simulink model "Eas_Integrated"  (R2021a)
settings: Solver=FixedStepDiscrete  StartTime=0.0  StopTime=inf  FixedStep=0.01  RelTol=1e-3
values from neighbouring files (symbols this model uses):
  Accelerator_Pedal_0 = 0.0    [DPF_Data_Dictionary.sldd]
  Adblue_Concentration_1 = 31.8    [Scr_Regeneration.sldd]
  Adblue_Concentration_2 = 33.2    [Scr_Regeneration.sldd]
  Adblue_Low_Level = 20.0    [Scr_Regeneration.sldd]
  Break_Pedal_0 = 0.0    [DPF_Data_Dictionary.sldd]
  Clutch_Pedal_0 = 0.0    [DPF_Data_Dictionary.sldd]
  Constant = 3.0    [Scr_Regeneration.sldd]
  Coolant_Temp_80 = 80.0    [DPF_Data_Dictionary.sldd]
  Crank_Angle_10 = 10.0    [DPF_Data_Dictionary.sldd]
  Crank_Angle_190 = 190.0    [DPF_Data_Dictionary.sldd]
  Crank_Angle_215 = 215.0    [DPF_Data_Dictionary.sldd]
  Crank_Angle_35 = 35.0    [DPF_Data_Dictionary.sldd]
  Crank_Angle_370 = 370.0    [DPF_Data_Dictionary.sldd]
  Crank_Angle_395 = 395.0    [DPF_Data_Dictionary.sldd]
  Crank_Angle_550 = 550.0    [DPF_Data_Dictionary.sldd]
  Crank_Angle_575 = 575.0    [DPF_Data_Dictionary.sldd]
  Dcrg_Press = 6.0    [Scr_Regeneration.sldd]
  DPF_Temp_Auto_250 = 250.0    [DPF_Data_Dictionary.sldd]
  DPF_Temp_Manual_200 = 200.0    [DPF_Data_Dictionary.sldd]
  Lamp_Off = 1.0    [Scr_Regeneration.sldd]
  Lamp_On = 0.0    [Scr_Regeneration.sldd]
  Nozzle_Area = 1.13E-6    [Scr_Regeneration.sldd]
  Nozzle_FlowRate = 0.099    [Scr_Regeneration.sldd]
  rpm_1500 = 1500.0    [DPF_Data_Dictionary.sldd]
  scr_temp200 = 200.0    [Scr_Regeneration.sldd]
  Soot_Deposition_Auto_80 = 80.0    [DPF_Data_Dictionary.sldd]
  Soot_Deposition_Manual_80 = 80.0    [DPF_Data_Dictionary.sldd]
  Soot_Deposition_Service_95 = 95.0    [DPF_Data_Dictionary.sldd]
  Tank_Condition = 0.0    [Scr_Regeneration.sldd]
  Var = 2.0    [Scr_Regeneration.sldd]
  Vehicle_Speed_55 = 55.0    [DPF_Data_Dictionary.sldd]
undefined symbols (not defined in the file or in its folder): adblue_capacity
libraries: simulink x2
settings Model: DataDictionary=DPF_Data_Dictionary.sldd  Creator=Admin  LastModifiedBy=SOMNATH
settings OptimizationCC: BlockReduction=off  DefaultParameterBehavior=Inlined  UseDivisionForNetSlopeComputation=on  EnhancedBackFolding=on  PassReuseOutputArgsAs=Individual arguments  EfficientFloat2IntCast=on  LifeSpan=Inf  OptimizeBlockOrder=speed  DifferentSizesBufferReuse=on  OptimizationCustomize=off  EfficientTunableParamExpr=on
settings DebuggingCC: SignalInfNanChecking=error  SignalRangeChecking=error  ReadBeforeWriteMsg=EnableAllAsError  WriteAfterWriteMsg=EnableAllAsError  WriteAfterReadMsg=EnableAllAsError  AlgebraicLoopMsg=error  ArtificialAlgebraicLoopMsg=error  SaveWithDisabledLinksMsg=error  SaveWithParameterizedLinksMsg=error  BlockPriorityViolationMsg=error  SolverPrmCheckMsg=error  InheritedTsInSrcMsg=error  SingleTaskRateTransMsg=error  TasksWithSamePriorityMsg=error  SigSpecEnsureSampleTimeMsg=error  CheckMatrixSingularityMsg=error  IntegerOverflowMsg=error  ParameterUnderflowMsg=error  ParameterPrecisionLossMsg=error  ParameterTunabilityLossMsg=error  UnderSpecifiedDataTypeMsg=error  UnnecessaryDatatypeConvMsg=warning  VectorMatrixConversionMsg=error  SignalLabelMismatchMsg=error  UnconnectedInputMsg=error  UnconnectedOutputMsg=error  UnconnectedLineMsg=error  SFcnCompatibilityMsg=error  UniqueDataStoreMsg=error  BusObjectLabelMismatch=error  RootOutportRequireBusObject=error  AssertControl=DisableAll  ModelReferenceIOMsg=error  ModelReferenceIOMismatchMessage=error  UnknownTsInhSupMsg=error  ModelReferenceDataLoggingMessage=error  StateNameClashWarn=warning  StrictBusMsg=ErrorOnBusTreatedAsVector  NonBusSignalsTreatedAsBus=error  SFInvalidInputDataAccessInChartInitDiag=error  SFTransitionOutsideNaturalParentDiag=error  SFUnreachableExecutionPathDiag=error  SFUndirectedBroadcastEventsDiag=error  SFTransitionActionBeforeConditionDiag=error  SFTemporalDelaySmallerThanSampleTimeDiag=error  SFSelfTransitionDiag=error  SFExecutionAtInitializationDiag=error  IntegerSaturationMsg=error
settings SFSimCC: CompileTimeRecursionLimit=0  EnableRuntimeRecursion=off  MATLABDynamicMemAlloc=off
settings RTWCC: SystemTargetFile=ert.tlc  GenCodeOnly=on  TemplateMakefile=ert_default_tmf  GenerateReport=on  Toolchain=MinGW64 | gmake (64-bit Windows)  IncludeHyperlinkInReport=on  LaunchReport=on  GenerateTraceInfo=on  GenerateTraceReport=on  GenerateTraceReportSl=on  GenerateTraceReportSf=on  GenerateTraceReportEml=on  GenerateWebview=on  GenerateCodeReplacementReport=on
settings CodeAppCC: ForceParamTrailComments=on  IgnoreCustomStorageClasses=off  OperatorAnnotations=on  SimulinkDataObjDesc=on  SFDataObjDesc=on  MATLABFcnDesc=on  MangleLength=4  InsertBlockDesc=on  ReqsInCode=on
settings ERTTargetCC: TargetLangStandard=C99 (ISO)  UtilityFuncGeneration=Shared location  GenerateSampleERTMain=on  IncludeMdlTerminateFcn=off  SuppressErrorStatus=on  SupportAbsoluteTime=off  SupportNonFinite=off  ParenthesesLevel=Maximum  CastingMode=Standards  GenerateSharedConstants=off  InlinedParameterPlacement=NonHierarchical  ERTCustomFileTemplate=example_file_process.tlc  PreserveExpressionOrder=on  EnableSignedLeftShifts=off  EnableSignedRightShifts=off
settings ConfigComp: CovMetricSettings=dcmwe  DVMode=PropertyProving  DVTestSuiteOptimization=Auto  DVDetectDeadLogic=on  DVDetectActiveLogic=on  DVDetectOutOfBounds=on  DVDetectInfNaN=on  DVDesignMinMaxCheck=on  DVDetectDSMAccessViolations=on  DVDetectHISMViolationsHisl_0002=on  DVDetectHISMViolationsHisl_0003=on  DVDetectHISMViolationsHisl_0004=on  DVDetectHISMViolationsHisl_0028=on  DVDetectBlockInputRangeViolations=on  DVSaveExpectedOutput=on  DVRandomizeNoEffectData=on  DVSaveHarnessModel=on

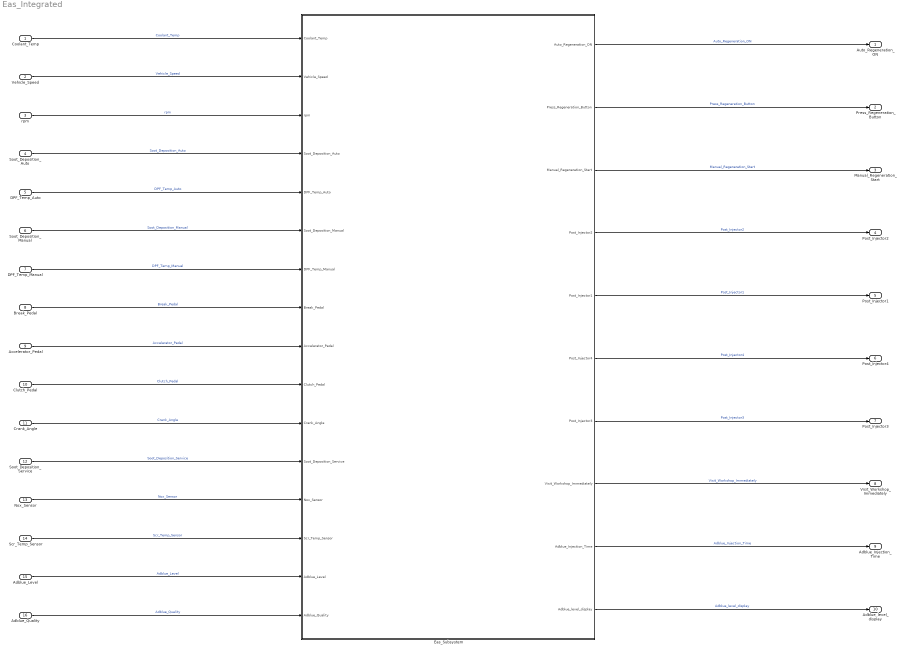
== system Eas_Integrated ==
  Coolant_Temp : Inport  OutDataTypeStr=int16
  Vehicle_Speed : Inport  Port=2  OutDataTypeStr=uint8
  rpm : Inport  Port=3  OutDataTypeStr=uint16
  Soot_Deposition_Auto : Inport  Port=4  OutDataTypeStr=uint8
  DPF_Temp_Auto : Inport  Port=5  OutDataTypeStr=uint8
  Soot_Deposition_Manual : Inport  Port=6  OutDataTypeStr=uint8
  DPF_Temp_Manual : Inport  Port=7  OutDataTypeStr=int16
  Break_Pedal : Inport  Port=8  OutDataTypeStr=boolean
  Accelerator_Pedal : Inport  Port=9  OutDataTypeStr=boolean
  Clutch_Pedal : Inport  Port=10  OutDataTypeStr=boolean
  Crank_Angle : Inport  Port=11  OutDataTypeStr=uint16
  Soot_Deposition_Service : Inport  Port=12  OutDataTypeStr=uint8
  Nox_Sensor : Inport  Port=13  OutDataTypeStr=uint16
  Scr_Temp_Sensor : Inport  Port=14  OutDataTypeStr=uint16
  Adblue_Level : Inport  Port=15  OutDataTypeStr=uint8
  Adblue_Quality : Inport  Port=16  OutDataTypeStr=double
  Eas_Subsystem : Subsystem  TreatAsAtomicUnit=on
  Auto_Regeneration_ON : Outport
  Press_Regeneration_Button : Outport  Port=2
  Manual_Regeneration_Start : Outport  Port=3
  Post_Injector2 : Outport  Port=4
  Post_Injector1 : Outport  Port=5
  Post_Injector4 : Outport  Port=6
  Post_Injector3 : Outport  Port=7
  Visit_Workshop_Immediately : Outport  Port=8
  Adblue_Injection_Time : Outport  Port=9  OutMin=0  OutMax=1500  OutDataTypeStr=double
  Adblue_level_display : Outport  Port=10  OutDataTypeStr=Enum: adblue_capacity
  wires:
  Eas_Subsystem/10(Adblue_level_display) -> Adblue_level_display/1  "Adblue_level_display"
  Eas_Subsystem/9(Adblue_Injection_Time) -> Adblue_Injection_Time/1  "Adblue_Injection_Time"
  Eas_Subsystem/7(Post_Injector3) -> Post_Injector3/1  "Post_Injector3"
  Eas_Subsystem/1(Auto_Regeneration_ON) -> Auto_Regeneration_ON/1  "Auto_Regeneration_ON"
  Eas_Subsystem/8(Visit_Workshop_Immediately) -> Visit_Workshop_Immediately/1  "Visit_Workshop_Immediately"
  Eas_Subsystem/6(Post_Injector4) -> Post_Injector4/1  "Post_Injector4"
  Eas_Subsystem/2(Press_Regeneration_Button) -> Press_Regeneration_Button/1  "Press_Regeneration_Button"
  Eas_Subsystem/5(Post_Injector1) -> Post_Injector1/1  "Post_Injector1"
  Eas_Subsystem/4(Post_Injector2) -> Post_Injector2/1  "Post_Injector2"
  Eas_Subsystem/3(Manual_Regeneration_Start) -> Manual_Regeneration_Start/1  "Manual_Regeneration_Start"
  Adblue_Quality/1 -> Eas_Subsystem/16(Adblue_Quality)  "Adblue_Quality"
  Adblue_Level/1 -> Eas_Subsystem/15(Adblue_Level)  "Adblue_Level"
  DPF_Temp_Auto/1 -> Eas_Subsystem/5(DPF_Temp_Auto)  "DPF_Temp_Auto"
  Accelerator_Pedal/1 -> Eas_Subsystem/9(Accelerator_Pedal)  "Accelerator_Pedal"
  Scr_Temp_Sensor/1 -> Eas_Subsystem/14(Scr_Temp_Sensor)  "Scr_Temp_Sensor"
  Nox_Sensor/1 -> Eas_Subsystem/13(Nox_Sensor)  "Nox_Sensor"
  Soot_Deposition_Service/1 -> Eas_Subsystem/12(Soot_Deposition_Service)  "Soot_Deposition_Service"
  Crank_Angle/1 -> Eas_Subsystem/11(Crank_Angle)  "Crank_Angle"
  Clutch_Pedal/1 -> Eas_Subsystem/10(Clutch_Pedal)  "Clutch_Pedal"
  Break_Pedal/1 -> Eas_Subsystem/8(Break_Pedal)  "Break_Pedal"
  DPF_Temp_Manual/1 -> Eas_Subsystem/7(DPF_Temp_Manual)  "DPF_Temp_Manual"
  Soot_Deposition_Manual/1 -> Eas_Subsystem/6(Soot_Deposition_Manual)  "Soot_Deposition_Manual"
  Soot_Deposition_Auto/1 -> Eas_Subsystem/4(Soot_Deposition_Auto)  "Soot_Deposition_Auto"
  rpm/1 -> Eas_Subsystem/3(rpm)  "rpm"
  Vehicle_Speed/1 -> Eas_Subsystem/2(Vehicle_Speed)  "Vehicle_Speed"
  Coolant_Temp/1 -> Eas_Subsystem/1(Coolant_Temp)  "Coolant_Temp"

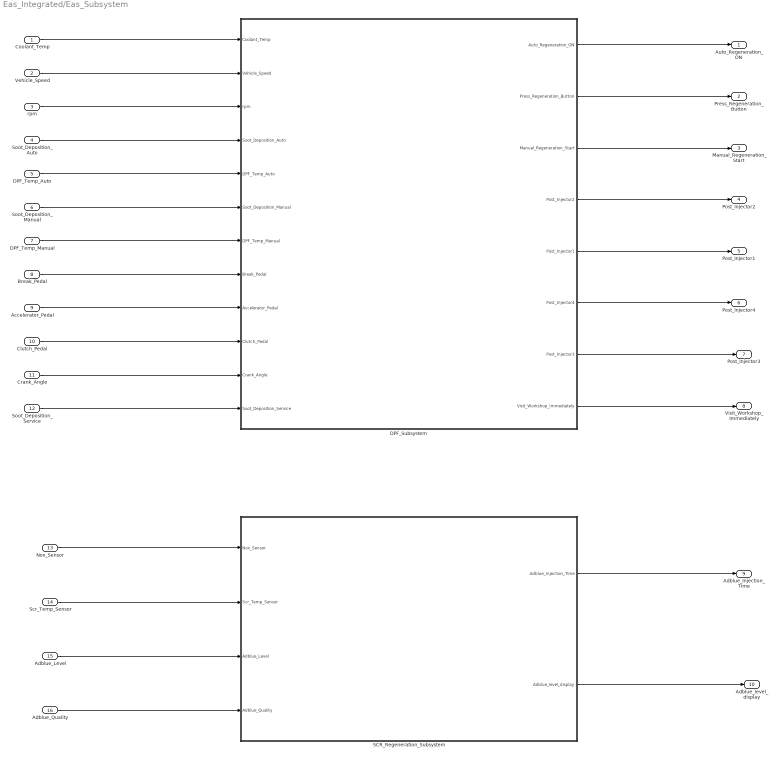
== system Eas_Integrated/Eas_Subsystem ==
  Coolant_Temp : Inport
  Vehicle_Speed : Inport  Port=2
  rpm : Inport  Port=3
  Soot_Deposition_Auto : Inport  Port=4
  DPF_Temp_Auto : Inport  Port=5
  Soot_Deposition_Manual : Inport  Port=6
  DPF_Temp_Manual : Inport  Port=7
  Break_Pedal : Inport  Port=8
  Accelerator_Pedal : Inport  Port=9
  Clutch_Pedal : Inport  Port=10
  Crank_Angle : Inport  Port=11
  Soot_Deposition_Service : Inport  Port=12
  Nox_Sensor : Inport  Port=13
  Scr_Temp_Sensor : Inport  Port=14
  Adblue_Level : Inport  Port=15  OutDataTypeStr=uint8
  Adblue_Quality : Inport  Port=16
  DPF_Subsystem : Subsystem  TreatAsAtomicUnit=on
  SCR_Regeneration_Subsystem : Subsystem  TreatAsAtomicUnit=on
  Auto_Regeneration_ON : Outport
  Press_Regeneration_Button : Outport  Port=2
  Manual_Regeneration_Start : Outport  Port=3
  Post_Injector2 : Outport  Port=4
  Post_Injector1 : Outport  Port=5
  Post_Injector4 : Outport  Port=6
  Post_Injector3 : Outport  Port=7
  Visit_Workshop_Immediately : Outport  Port=8
  Adblue_Injection_Time : Outport  Port=9
  Adblue_level_display : Outport  Port=10
  wires:
  Vehicle_Speed/1 -> DPF_Subsystem/2(Vehicle_Speed)
  SCR_Regeneration_Subsystem/1(Adblue_Injection_Time) -> Adblue_Injection_Time/1
  Accelerator_Pedal/1 -> DPF_Subsystem/9(Accelerator_Pedal)
  DPF_Temp_Manual/1 -> DPF_Subsystem/7(DPF_Temp_Manual)
  rpm/1 -> DPF_Subsystem/3(rpm)
  DPF_Temp_Auto/1 -> DPF_Subsystem/5(DPF_Temp_Auto)
  DPF_Subsystem/2(Press_Regeneration_Button) -> Press_Regeneration_Button/1
  Crank_Angle/1 -> DPF_Subsystem/11(Crank_Angle)
  Scr_Temp_Sensor/1 -> SCR_Regeneration_Subsystem/2(Scr_Temp_Sensor)
  Soot_Deposition_Auto/1 -> DPF_Subsystem/4(Soot_Deposition_Auto)
  DPF_Subsystem/5(Post_Injector1) -> Post_Injector1/1
  Soot_Deposition_Service/1 -> DPF_Subsystem/12(Soot_Deposition_Service)
  Soot_Deposition_Manual/1 -> DPF_Subsystem/6(Soot_Deposition_Manual)
  Adblue_Quality/1 -> SCR_Regeneration_Subsystem/4(Adblue_Quality)
  Clutch_Pedal/1 -> DPF_Subsystem/10(Clutch_Pedal)
  DPF_Subsystem/3(Manual_Regeneration_Start) -> Manual_Regeneration_Start/1
  Break_Pedal/1 -> DPF_Subsystem/8(Break_Pedal)
  DPF_Subsystem/7(Post_Injector3) -> Post_Injector3/1
  DPF_Subsystem/6(Post_Injector4) -> Post_Injector4/1
  Coolant_Temp/1 -> DPF_Subsystem/1(Coolant_Temp)
  DPF_Subsystem/8(Visit_Workshop_Immediately) -> Visit_Workshop_Immediately/1
  Nox_Sensor/1 -> SCR_Regeneration_Subsystem/1(Nox_Sensor)
  DPF_Subsystem/1(Auto_Regeneration_ON) -> Auto_Regeneration_ON/1
  DPF_Subsystem/4(Post_Injector2) -> Post_Injector2/1
  SCR_Regeneration_Subsystem/2(Adblue_level_display) -> Adblue_level_display/1
  Adblue_Level/1 -> SCR_Regeneration_Subsystem/3(Adblue_Level)

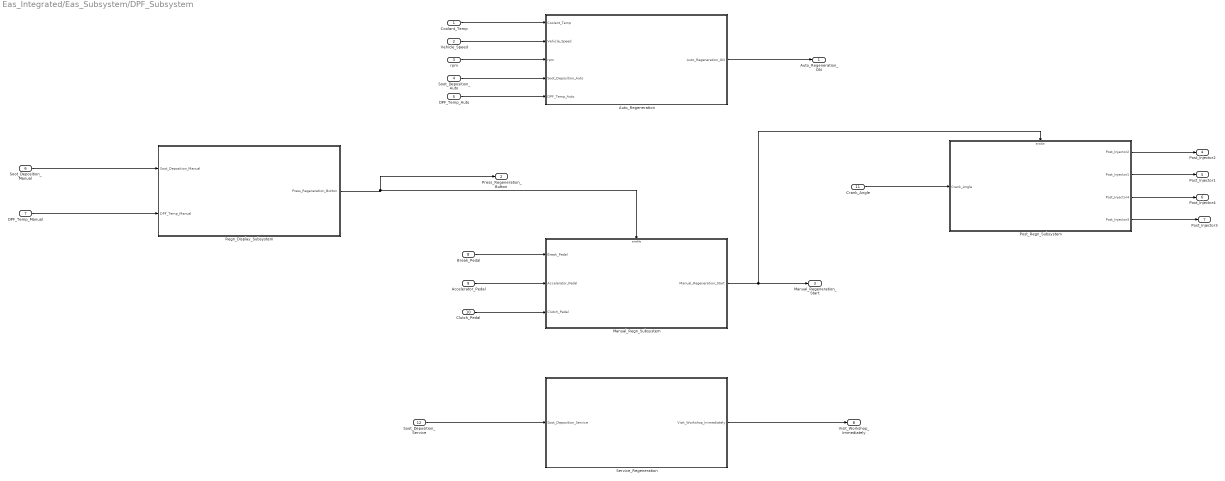
== system Eas_Integrated/Eas_Subsystem/DPF_Subsystem ==
  Coolant_Temp : Inport
  Vehicle_Speed : Inport  Port=2
  rpm : Inport  Port=3
  Soot_Deposition_Auto : Inport  Port=4
  DPF_Temp_Auto : Inport  Port=5
  Soot_Deposition_Manual : Inport  Port=6
  DPF_Temp_Manual : Inport  Port=7
  Break_Pedal : Inport  Port=8
  Accelerator_Pedal : Inport  Port=9
  Clutch_Pedal : Inport  Port=10
  Crank_Angle : Inport  Port=11
  Soot_Deposition_Service : Inport  Port=12
  Auto_Regeneration : Subsystem  TreatAsAtomicUnit=on
  Manual_Regn_Subsystem : Subsystem  TreatAsAtomicUnit=on
  Post_Regn_Subsystem : Subsystem
  Regn_Display_Subsystem : Subsystem
  Service_Regeneration : Subsystem
  Auto_Regeneration_ON : Outport
  Press_Regeneration_Button : Outport  Port=2
  Manual_Regeneration_Start : Outport  Port=3
  Post_Injector2 : Outport  Port=4
  Post_Injector1 : Outport  Port=5
  Post_Injector4 : Outport  Port=6
  Post_Injector3 : Outport  Port=7
  Visit_Workshop_Immediately : Outport  Port=8
  wires:
  Soot_Deposition_Auto/1 -> Auto_Regeneration/4(Soot_Deposition_Auto)
  Auto_Regeneration/1(Auto_Regeneration_ON) -> Auto_Regeneration_ON/1
  Coolant_Temp/1 -> Auto_Regeneration/1(Coolant_Temp)
  rpm/1 -> Auto_Regeneration/3(rpm)
  Vehicle_Speed/1 -> Auto_Regeneration/2(Vehicle_Speed)
  DPF_Temp_Auto/1 -> Auto_Regeneration/5(DPF_Temp_Auto)
  Crank_Angle/1 -> Post_Regn_Subsystem/1(Crank_Angle)
  Post_Regn_Subsystem/2(Post_Injector1) -> Post_Injector1/1
  Post_Regn_Subsystem/3(Post_Injector4) -> Post_Injector4/1
  Manual_Regn_Subsystem/1(Manual_Regeneration_Start) -> Manual_Regeneration_Start/1, Post_Regn_Subsystem/Enable
  Post_Regn_Subsystem/4(Post_Injector3) -> Post_Injector3/1
  Soot_Deposition_Manual/1 -> Regn_Display_Subsystem/1(Soot_Deposition_Manual)
  DPF_Temp_Manual/1 -> Regn_Display_Subsystem/2(DPF_Temp_Manual)
  Regn_Display_Subsystem/1(Press_Regeneration_Button) -> Manual_Regn_Subsystem/Enable, Press_Regeneration_Button/1
  Post_Regn_Subsystem/1(Post_Injector2) -> Post_Injector2/1
  Accelerator_Pedal/1 -> Manual_Regn_Subsystem/2(Accelerator_Pedal)
  Clutch_Pedal/1 -> Manual_Regn_Subsystem/3(Clutch_Pedal)
  Break_Pedal/1 -> Manual_Regn_Subsystem/1(Break_Pedal)
  Soot_Deposition_Service/1 -> Service_Regeneration/1(Soot_Deposition_Service)
  Service_Regeneration/1(Visit_Workshop_Immediately) -> Visit_Workshop_Immediately/1

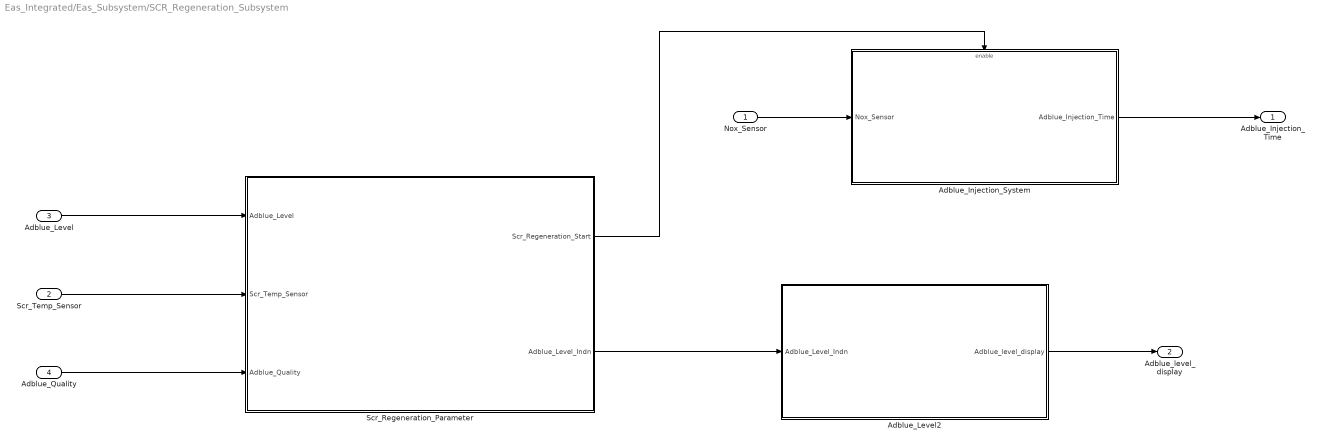
== system Eas_Integrated/Eas_Subsystem/SCR_Regeneration_Subsystem ==
  Nox_Sensor : Inport
  Scr_Temp_Sensor : Inport  Port=2
  Adblue_Level : Inport  Port=3  OutDataTypeStr=uint8
  Adblue_Quality : Inport  Port=4
  Adblue_Injection_System : Subsystem  Tag=Adblue_Injection_System
      settings: AttributesFormatString=%<Description>
  Adblue_Level2 : Subsystem  Tag=Adblue_Level2  Description=|  TreatAsAtomicUnit=on
      | This subsystem models a digital thermometer composed of a simple
      | temperature sensor and an ADC.
      settings: AttributesFormatString=%<Description>
  Scr_Regeneration_Parameter : Subsystem  Tag=Scr_Regeneration_Parameter  Description=|  TreatAsAtomicUnit=on
      | This subsystem models a digital thermometer composed of a simple
      | temperature sensor and an ADC.
      settings: AttributesFormatString=%<BlockDescription>
  Adblue_Injection_Time : Outport
  Adblue_level_display : Outport  Port=2
  wires:
  Scr_Regeneration_Parameter/1(Scr_Regeneration_Start) -> Adblue_Injection_System/Enable
  Adblue_Injection_System/1(Adblue_Injection_Time) -> Adblue_Injection_Time/1
  Scr_Temp_Sensor/1 -> Scr_Regeneration_Parameter/2(Scr_Temp_Sensor)
  Adblue_Level/1 -> Scr_Regeneration_Parameter/1(Adblue_Level)
  Scr_Regeneration_Parameter/2(Adblue_Level_Indn) -> Adblue_Level2/1(Adblue_Level_Indn)
  Nox_Sensor/1 -> Adblue_Injection_System/1(Nox_Sensor)
  Adblue_Level2/1(Adblue_level_display) -> Adblue_level_display/1
  Adblue_Quality/1 -> Scr_Regeneration_Parameter/3(Adblue_Quality)

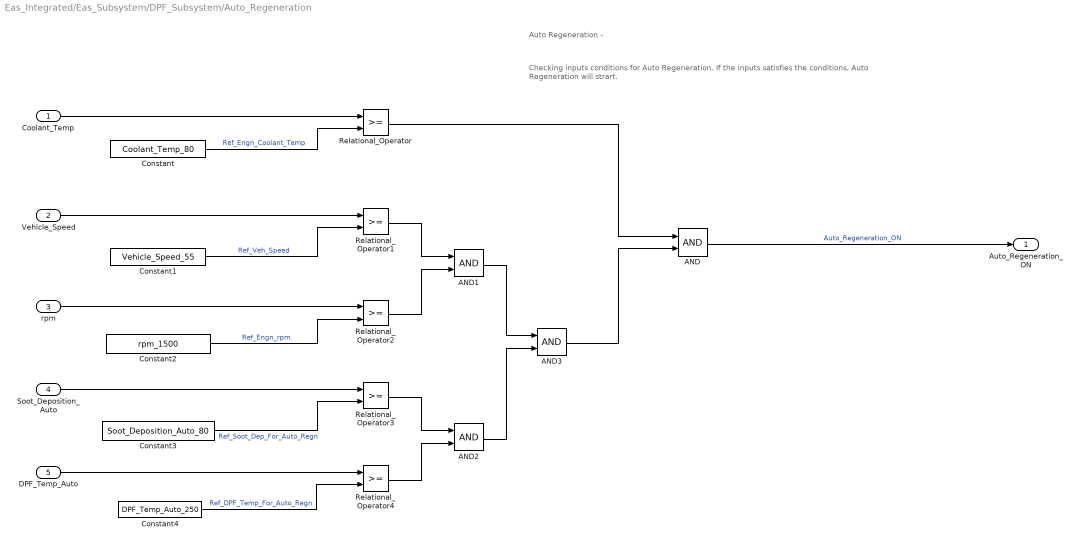
== system Eas_Integrated/Eas_Subsystem/DPF_Subsystem/Auto_Regeneration ==
  note: Auto Regeneration -
  note: Checking inputs conditions for Auto Regeneration. If the inputs satisfies the conditions, Auto Regeneration will strart.
  Coolant_Temp : Inport
  Vehicle_Speed : Inport  Port=2
  rpm : Inport  Port=3
  Soot_Deposition_Auto : Inport  Port=4
  DPF_Temp_Auto : Inport  Port=5
  AND{,1..3} (4 alike) : Logic  AllPortsSameDT=off  OutDataTypeStr=boolean
  Constant : Constant  Value=Coolant_Temp_80
  Constant1 : Constant  Value=Vehicle_Speed_55
  Constant2 : Constant  Value=rpm_1500
  Constant3 : Constant  Value=Soot_Deposition_Auto_80
  Constant4 : Constant  Value=DPF_Temp_Auto_250
  Relational_Operator{,1..4} (5 alike) : RelationalOperator  RndMeth=Simplest
  Auto_Regeneration_ON : Outport
  wires:
  DPF_Temp_Auto/1 -> Relational_Operator4/1
  Soot_Deposition_Auto/1 -> Relational_Operator3/1
  Vehicle_Speed/1 -> Relational_Operator1/1
  rpm/1 -> Relational_Operator2/1
  AND/1 -> Auto_Regeneration_ON/1  "Auto_Regeneration_ON"
  Constant/1 -> Relational_Operator/2  "Ref_Engn_Coolant_Temp"
  Constant1/1 -> Relational_Operator1/2  "Ref_Veh_Speed"
  Constant2/1 -> Relational_Operator2/2  "Ref_Engn_rpm"
  Constant3/1 -> Relational_Operator3/2  "Ref_Soot_Dep_For_Auto_Regn"
  Constant4/1 -> Relational_Operator4/2  "Ref_DPF_Temp_For_Auto_Regn"
  Relational_Operator1/1 -> AND1/1
  Relational_Operator2/1 -> AND1/2
  Relational_Operator3/1 -> AND2/1
  Relational_Operator4/1 -> AND2/2
  Relational_Operator/1 -> AND/1
  AND1/1 -> AND3/1
  AND2/1 -> AND3/2
  AND3/1 -> AND/2
  Coolant_Temp/1 -> Relational_Operator/1

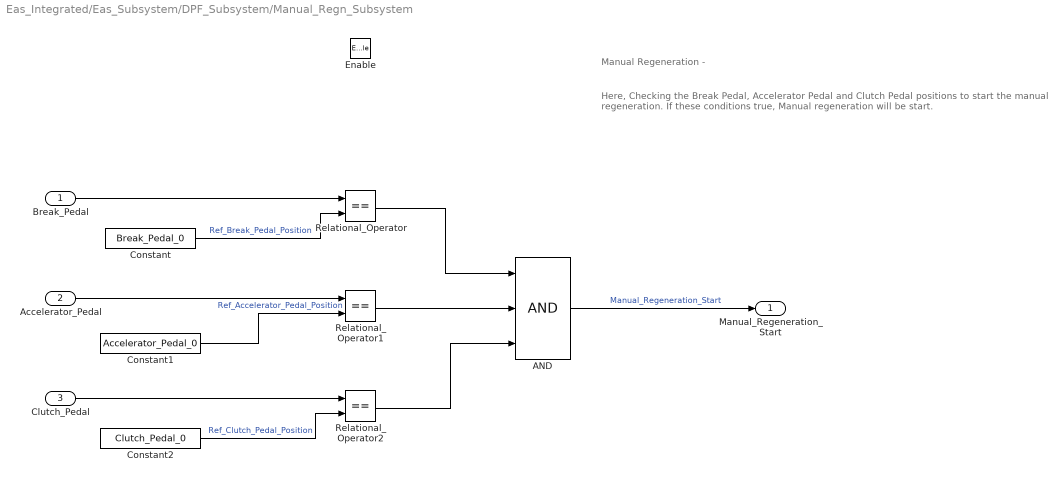
== system Eas_Integrated/Eas_Subsystem/DPF_Subsystem/Manual_Regn_Subsystem ==
  note: Here, Checking the Break Pedal, Accelerator Pedal and Clutch Pedal positions to start the manual regeneration. If these conditions true, Manual regeneration will be start.
  note: Manual Regeneration -
  Break_Pedal : Inport
  Accelerator_Pedal : Inport  Port=2
  Clutch_Pedal : Inport  Port=3
  Enable : EnablePort
  AND : Logic  Inputs=3  AllPortsSameDT=off  OutDataTypeStr=boolean
  Constant : Constant  Value=Break_Pedal_0
  Constant1 : Constant  Value=Accelerator_Pedal_0
  Constant2 : Constant  Value=Clutch_Pedal_0
  Relational_Operator : RelationalOperator  Operator===  RndMeth=Simplest
  Relational_Operator1 : RelationalOperator  Operator===  RndMeth=Simplest
  Relational_Operator2 : RelationalOperator  Operator===  RndMeth=Simplest
  Manual_Regeneration_Start : Outport
  wires:
  Constant/1 -> Relational_Operator/2  "Ref_Break_Pedal_Position"
  Break_Pedal/1 -> Relational_Operator/1
  Accelerator_Pedal/1 -> Relational_Operator1/1
  Constant1/1 -> Relational_Operator1/2  "Ref_Accelerator_Pedal_Position"
  Constant2/1 -> Relational_Operator2/2  "Ref_Clutch_Pedal_Position"
  Clutch_Pedal/1 -> Relational_Operator2/1
  Relational_Operator1/1 -> AND/2
  Relational_Operator/1 -> AND/1
  Relational_Operator2/1 -> AND/3
  AND/1 -> Manual_Regeneration_Start/1  "Manual_Regeneration_Start"

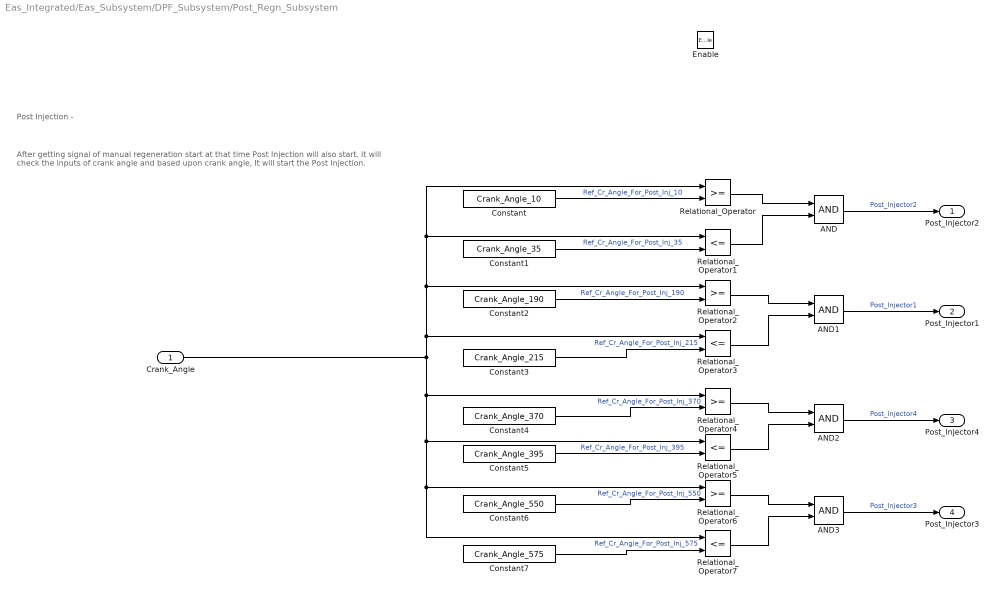
== system Eas_Integrated/Eas_Subsystem/DPF_Subsystem/Post_Regn_Subsystem ==
  note: After getting signal of manual regeneration start at that time Post Injection will also start. It will check the inputs of crank angle and based upon crank angle, It will start the Post Injection.
  note: Post Injection -
  Crank_Angle : Inport
  Enable : EnablePort
  AND{,1..3} (4 alike) : Logic  AllPortsSameDT=off  OutDataTypeStr=boolean
  Constant : Constant  Value=Crank_Angle_10
  Constant1 : Constant  Value=Crank_Angle_35
  Constant2 : Constant  Value=Crank_Angle_190
  Constant3 : Constant  Value=Crank_Angle_215
  Constant4 : Constant  Value=Crank_Angle_370
  Constant5 : Constant  Value=Crank_Angle_395
  Constant6 : Constant  Value=Crank_Angle_550
  Constant7 : Constant  Value=Crank_Angle_575
  Relational_Operator{,2,4,6} (4 alike) : RelationalOperator  OutDataTypeStr=boolean  RndMeth=Simplest
  Relational_Operator{1,3,5,7} (4 alike) : RelationalOperator  Operator=<=  OutDataTypeStr=boolean  RndMeth=Simplest
  Post_Injector2 : Outport
  Post_Injector1 : Outport  Port=2
  Post_Injector4 : Outport  Port=3
  Post_Injector3 : Outport  Port=4
  wires:
  Constant3/1 -> Relational_Operator3/2  "Ref_Cr_Angle_For_Post_Inj_215"
  Crank_Angle/1 -> Relational_Operator4/1, Relational_Operator5/1, Relational_Operator6/1, Relational_Operator7/1, Relational_Operator3/1, Relational_Operator2/1, Relational_Operator1/1, Relational_Operator/1
  Constant5/1 -> Relational_Operator5/2  "Ref_Cr_Angle_For_Post_Inj_395"
  Relational_Operator6/1 -> AND3/1
  Constant/1 -> Relational_Operator/2  "Ref_Cr_Angle_For_Post_Inj_10"
  Constant6/1 -> Relational_Operator6/2  "Ref_Cr_Angle_For_Post_Inj_550"
  Relational_Operator7/1 -> AND3/2
  Relational_Operator5/1 -> AND2/2
  Relational_Operator2/1 -> AND1/1
  Relational_Operator4/1 -> AND2/1
  Relational_Operator1/1 -> AND/2
  Relational_Operator/1 -> AND/1
  Relational_Operator3/1 -> AND1/2
  Constant2/1 -> Relational_Operator2/2  "Ref_Cr_Angle_For_Post_Inj_190"
  Constant7/1 -> Relational_Operator7/2  "Ref_Cr_Angle_For_Post_Inj_575"
  Constant1/1 -> Relational_Operator1/2  "Ref_Cr_Angle_For_Post_Inj_35"
  AND1/1 -> Post_Injector1/1  "Post_Injector1"
  Constant4/1 -> Relational_Operator4/2  "Ref_Cr_Angle_For_Post_Inj_370"
  AND2/1 -> Post_Injector4/1  "Post_Injector4"
  AND/1 -> Post_Injector2/1  "Post_Injector2"
  AND3/1 -> Post_Injector3/1  "Post_Injector3"

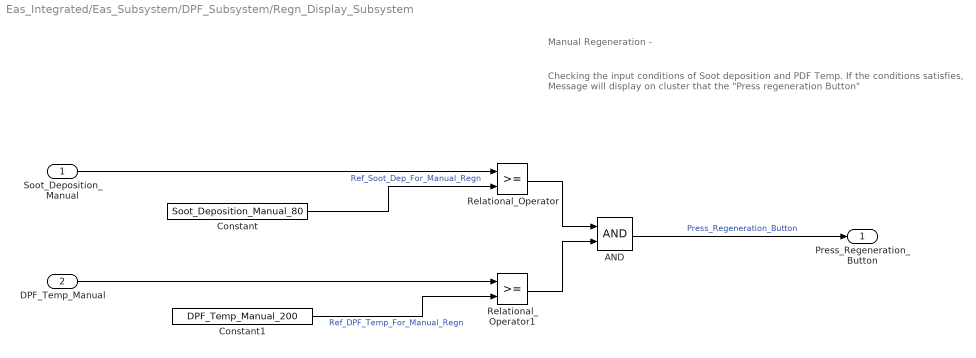
== system Eas_Integrated/Eas_Subsystem/DPF_Subsystem/Regn_Display_Subsystem ==
  note: Checking the input conditions of Soot deposition and PDF Temp. If the conditions satisfies, Message will display on cluster that the "Press regeneration Button"
  note: Manual Regeneration -
  Soot_Deposition_Manual : Inport
  DPF_Temp_Manual : Inport  Port=2
  AND : Logic  AllPortsSameDT=off  OutDataTypeStr=boolean
  Constant : Constant  Value=Soot_Deposition_Manual_80
  Constant1 : Constant  Value=DPF_Temp_Manual_200
  Relational_Operator : RelationalOperator  OutDataTypeStr=boolean  RndMeth=Simplest
  Relational_Operator1 : RelationalOperator  OutDataTypeStr=boolean  RndMeth=Simplest
  Press_Regeneration_Button : Outport
  wires:
  AND/1 -> Press_Regeneration_Button/1  "Press_Regeneration_Button"
  Soot_Deposition_Manual/1 -> Relational_Operator/1
  Constant1/1 -> Relational_Operator1/2  "Ref_DPF_Temp_For_Manual_Regn"
  Relational_Operator1/1 -> AND/2
  DPF_Temp_Manual/1 -> Relational_Operator1/1
  Relational_Operator/1 -> AND/1
  Constant/1 -> Relational_Operator/2  "Ref_Soot_Dep_For_Manual_Regn"

== system Eas_Integrated/Eas_Subsystem/DPF_Subsystem/Service_Regeneration ==
  note: Checking the inputs of Soot Deposition value, If the condition is geeting true,
      | Message will be show on cluster that the "Visit Worksop Immediately and It will send signal to ICU for torque reduction.
  note: Service Regeneration -
  Soot_Deposition_Service : Inport
  Constant3 : Constant  Value=Soot_Deposition_Service_95
  Relational_Operator3 : RelationalOperator  OutDataTypeStr=boolean  RndMeth=Simplest
  Visit_Workshop_Immediately : Outport
  wires:
  Constant3/1 -> Relational_Operator3/2  "Ref_Soot_Dep_For_Servc_Regn_95"
  Relational_Operator3/1 -> Visit_Workshop_Immediately/1  "Visit_Workshop_Immediately"
  Soot_Deposition_Service/1 -> Relational_Operator3/1

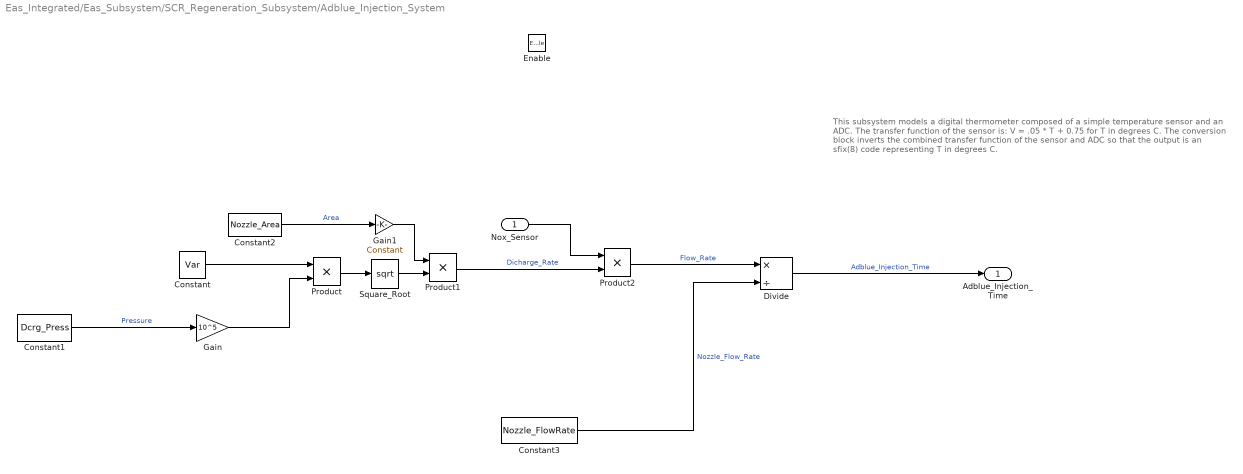
== system Eas_Integrated/Eas_Subsystem/SCR_Regeneration_Subsystem/Adblue_Injection_System ==
  note: This subsystem models a digital thermometer composed of a simple
      | temperature sensor and an ADC.  The transfer function of the sensor is:
      | V = .05 * T + 0.75
      | for T in degrees C.
      |
      | The conversion block inverts the combined transfer function of the sensor
      | and ADC so that the output is an sfix(8) code representing T in degrees C.
  Nox_Sensor : Inport  OutDataTypeStr=uint16
  Enable : EnablePort
  Constant : Constant  Value=Var
  Constant1 : Constant  Value=Dcrg_Press  OutDataTypeStr=int16
  Constant2 : Constant  Value=Nozzle_Area
  Constant3 : Constant  Value=Nozzle_FlowRate  OutDataTypeStr=double
  Divide : Product  Inputs=*/  OutDataTypeStr=Inherit: Inherit via back propagation
  Gain : Gain  Gain=10^5  ParamDataTypeStr=Inherit: Inherit from 'Gain'  OutDataTypeStr=double
  Gain1 : Gain  Gain=Constant
  Product : Product
  Product1 : Product
  Product2 : Product
  Square_Root : Sqrt  IntermediateResultsDataTypeStr=Inherit: Inherit from input
  Adblue_Injection_Time : Outport  OutDataTypeStr=double
  wires:
  Constant2/1 -> Gain1/1  "Area"
  Constant/1 -> Product/1
  Square_Root/1 -> Product1/2
  Product/1 -> Square_Root/1
  Constant1/1 -> Gain/1  "Pressure"
  Product2/1 -> Divide/1  "Flow_Rate"
  Gain1/1 -> Product1/1
  Divide/1 -> Adblue_Injection_Time/1  "Adblue_Injection_Time"
  Constant3/1 -> Divide/2  "Nozzle_Flow_Rate"
  Product1/1 -> Product2/2  "Dicharge_Rate"
  Nox_Sensor/1 -> Product2/1
  Gain/1 -> Product/2

== system Eas_Integrated/Eas_Subsystem/SCR_Regeneration_Subsystem/Adblue_Level2 ==
  note: This subsystem models a digital thermometer composed of a simple
      | temperature sensor and an ADC.  The transfer function of the sensor is:
      | V = .05 * T + 0.75
      | for T in degrees C.
      |
      | The conversion block inverts the combined transfer function of the sensor
      | and ADC so that the output is an sfix(8) code representing T in degrees C.
  Adblue_Level_Indn : Inport  OutDataTypeStr=boolean
  Enumerated_Constant : simulink/Sources/Enumerated Constant  OutDataTypeStr=Enum: adblue_capacity  Value=adblue_capacity.Adblue_Level_Low  SampleTime=inf
  Enumerated_Constant1 : simulink/Sources/Enumerated Constant  OutDataTypeStr=Enum: adblue_capacity  Value=adblue_capacity.Adblue_Level_high  SampleTime=inf
  Relational_Operator1 : RelationalOperator  Operator===  OutDataTypeStr=boolean  RndMeth=Simplest
  Switch2 : Switch  Criteria=u2 ~= 0  OutDataTypeStr=Inherit: Inherit via back propagation
  Tank_Condition : Constant  Value=Tank_Condition
  Adblue_level_display : Outport  OutDataTypeStr=Enum: adblue_capacity  VectorParamsAs1DForOutWhenUnconnected=off
  wires:
  Enumerated_Constant/1 -> Switch2/1
  Adblue_Level_Indn/1 -> Relational_Operator1/1
  Tank_Condition/1 -> Relational_Operator1/2  "Tank_Condition"
  Enumerated_Constant1/1 -> Switch2/3
  Relational_Operator1/1 -> Switch2/2
  Switch2/1 -> Adblue_level_display/1  "Adblue_level_display"

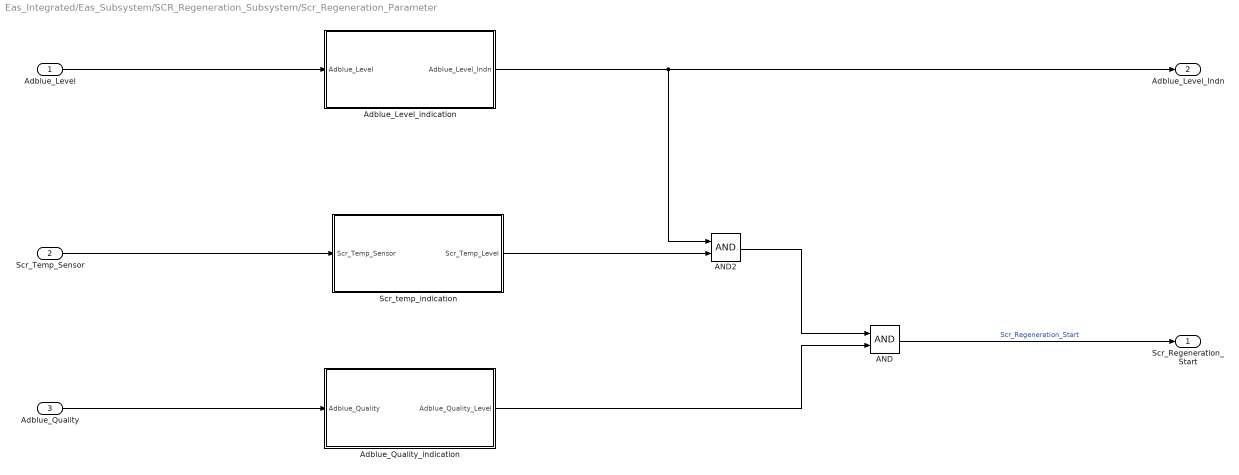
== system Eas_Integrated/Eas_Subsystem/SCR_Regeneration_Subsystem/Scr_Regeneration_Parameter ==
  Adblue_Level : Inport  OutDataTypeStr=uint8
  Scr_Temp_Sensor : Inport  Port=2  OutDataTypeStr=uint16
  Adblue_Quality : Inport  Port=3
  AND : Logic  AllPortsSameDT=off  OutDataTypeStr=boolean
  AND2 : Logic  AllPortsSameDT=off  OutDataTypeStr=boolean
  Adblue_Level_indication : Subsystem  Description=|  TreatAsAtomicUnit=on
      | This subsystem models a digital thermometer composed of a simple 
      | temperature sensor and an ADC.  The transfer function of the sensor is:
      | V = .05 * T + 0.75
      | for T in degrees C.  
      | 
      | The conversion block inverts the combined transfer function of the sensor 
      | and ADC so that the output is an sfix(8) code representing T in degrees C.
      settings: AttributesFormatString=%<BlockDescription>
  Adblue_Quality_indication : Subsystem  Description=|  TreatAsAtomicUnit=on
      | This subsystem models a digital thermometer composed of a simple 
      | temperature sensor and an ADC.  The transfer function of the sensor is:
      | V = .05 * T + 0.75
      | for T in degrees C.  
      | 
      | The conversion block inverts the combined transfer function of the sensor 
      | and ADC so that the output is an sfix(8) code representing T in degrees C.
      settings: AttributesFormatString=%<BlockDescription>
  Scr_temp_indication : Subsystem  Description=|  TreatAsAtomicUnit=on
      | This subsystem models a digital thermometer composed of a simple 
      | temperature sensor and an ADC.  The transfer function of the sensor is:
      | V = .05 * T + 0.75
      | for T in degrees C.  
      | 
      | The conversion block inverts the combined transfer function of the sensor 
      | and ADC so that the output is an sfix(8) code representing T in degrees C.
      settings: AttributesFormatString=%<BlockDescription>
  Scr_Regeneration_Start : Outport  OutDataTypeStr=boolean
  Adblue_Level_Indn : Outport  Port=2  OutDataTypeStr=boolean
  wires:
  Scr_Temp_Sensor/1 -> Scr_temp_indication/1(Scr_Temp_Sensor)
  Adblue_Quality_indication/1(Adblue_Quality_Level) -> AND/2
  Adblue_Quality/1 -> Adblue_Quality_indication/1(Adblue_Quality)
  Adblue_Level/1 -> Adblue_Level_indication/1(Adblue_Level)
  Adblue_Level_indication/1(Adblue_Level_Indn) -> AND2/1, Adblue_Level_Indn/1
  AND2/1 -> AND/1
  AND/1 -> Scr_Regeneration_Start/1  "Scr_Regeneration_Start"
  Scr_temp_indication/1(Scr_Temp_Level) -> AND2/2

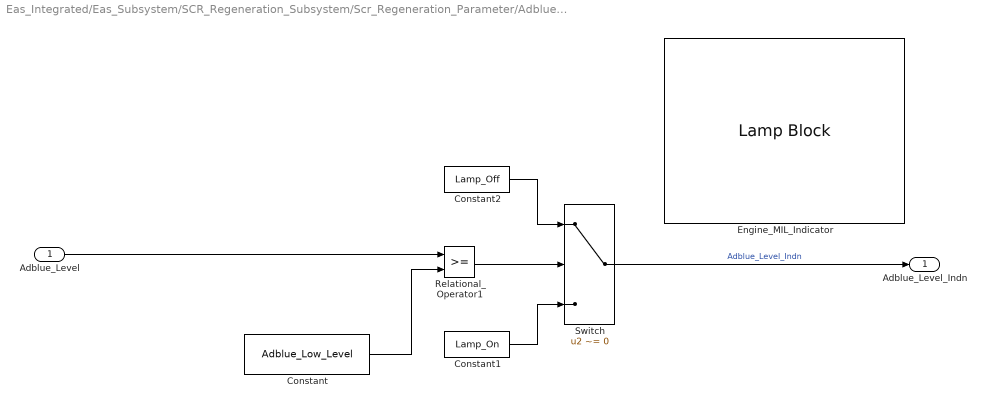
== system Eas_Integrated/Eas_Subsystem/SCR_Regeneration_Subsystem/Scr_Regeneration_Parameter/Adblue_Level_indication ==
  Adblue_Level : Inport  OutDataTypeStr=uint8
  Constant : Constant  Value=Adblue_Low_Level
  Constant1 : Constant  Value=Lamp_On
  Constant2 : Constant  Value=Lamp_Off
  Engine_MIL_Indicator : LampBlock  Icon=CheckEngine2
  Relational_Operator1 : RelationalOperator  OutDataTypeStr=boolean  RndMeth=Simplest
  Switch : Switch  Criteria=u2 ~= 0
  Adblue_Level_Indn : Outport
  wires:
  Adblue_Level/1 -> Relational_Operator1/1
  Constant/1 -> Relational_Operator1/2
  Switch/1 -> Adblue_Level_Indn/1  "Adblue_Level_Indn"
  Relational_Operator1/1 -> Switch/2
  Constant2/1 -> Switch/1
  Constant1/1 -> Switch/3

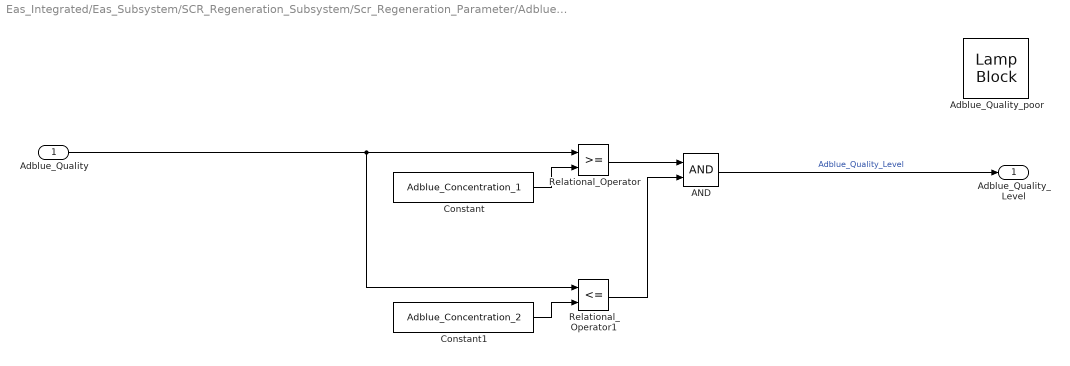
== system Eas_Integrated/Eas_Subsystem/SCR_Regeneration_Subsystem/Scr_Regeneration_Parameter/Adblue_Quality_indication ==
  Adblue_Quality : Inport  OutDataTypeStr=double
  AND : Logic  AllPortsSameDT=off  OutDataTypeStr=boolean
  Adblue_Quality_poor : LampBlock  Icon=Engine
  Constant : Constant  Value=Adblue_Concentration_1
  Constant1 : Constant  Value=Adblue_Concentration_2
  Relational_Operator : RelationalOperator  OutDataTypeStr=boolean  RndMeth=Simplest
  Relational_Operator1 : RelationalOperator  Operator=<=  OutDataTypeStr=boolean  RndMeth=Simplest
  Adblue_Quality_Level : Outport
  wires:
  Relational_Operator1/1 -> AND/2
  AND/1 -> Adblue_Quality_Level/1  "Adblue_Quality_Level"
  Relational_Operator/1 -> AND/1
  Constant/1 -> Relational_Operator/2
  Adblue_Quality/1 -> Relational_Operator1/1, Relational_Operator/1
  Constant1/1 -> Relational_Operator1/2

== system Eas_Integrated/Eas_Subsystem/SCR_Regeneration_Subsystem/Scr_Regeneration_Parameter/Scr_temp_indication ==
  Scr_Temp_Sensor : Inport  OutDataTypeStr=uint16
  Constant1 : Constant  Value=On
  Constant2 : Constant  Value=Off
  Relational_Operator : RelationalOperator  OutDataTypeStr=boolean  RndMeth=Simplest
  Switch : Switch  Criteria=u2 ~= 0
  scr_temp : Constant  Value=scr_temp200
  Scr_Temp_Level : Outport
  wires:
  Scr_Temp_Sensor/1 -> Relational_Operator/1
  Relational_Operator/1 -> Switch/2
  Constant1/1 -> Switch/1
  Constant2/1 -> Switch/3
  scr_temp/1 -> Relational_Operator/2  "scr_temp200"
  Switch/1 -> Scr_Temp_Level/1  "Scr_Temp_Level"
